simulink model "number"  (R2018a)
settings: Solver=VariableStepAuto  StartTime=0.0  StopTime=10.0  RelTol=1e-3
libraries: simulink_extras x32
settings Model: Creator=Edoardo Debenedetti  LastModifiedBy=Edoardo Debenedetti

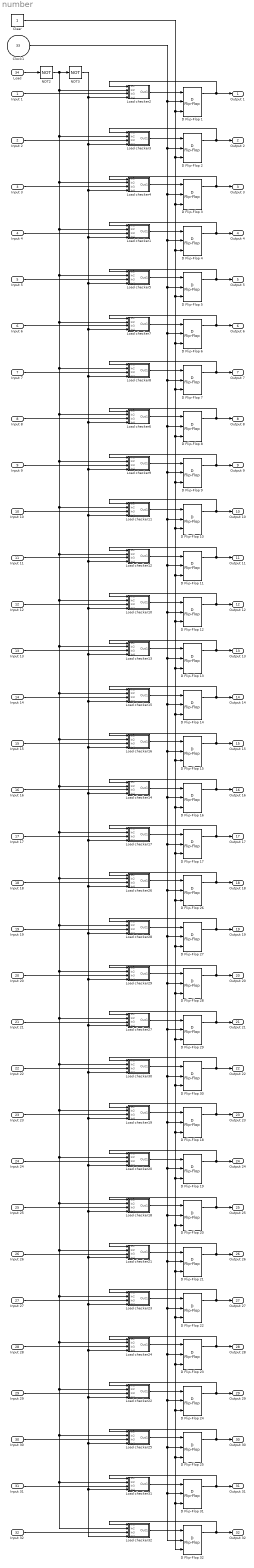
== system number ==
  Input 1 : Inport
  Input 2 : Inport  Port=2
  Input 3 : Inport  Port=3
  Input 4 : Inport  Port=4
  Input 5 : Inport  Port=5
  Input 6 : Inport  Port=6
  Input 7 : Inport  Port=7
  Input 8 : Inport  Port=8
  Input 9 : Inport  Port=9
  Input 10 : Inport  Port=10
  Input 11 : Inport  Port=11
  Input 12 : Inport  Port=12
  Input 13 : Inport  Port=13
  Input 14 : Inport  Port=14
  Input 15 : Inport  Port=15
  Input 16 : Inport  Port=16
  Input 17 : Inport  Port=17
  Input 18 : Inport  Port=18
  Input 19 : Inport  Port=19
  Input 20 : Inport  Port=20
  Input 21 : Inport  Port=21
  Input 22 : Inport  Port=22
  Input 23 : Inport  Port=23
  Input 24 : Inport  Port=24
  Input 25 : Inport  Port=25
  Input 26 : Inport  Port=26
  Input 27 : Inport  Port=27
  Input 28 : Inport  Port=28
  Input 29 : Inport  Port=29
  Input 30 : Inport  Port=30
  Input 31 : Inport  Port=31
  Input 32 : Inport  Port=32
  Clock1 : Inport  Port=33
  Load : Inport  Port=34
  Clear : Constant
  D Flip-Flop {1..32} (32 alike) : simulink_extras/Flip Flops/D Flip-Flop
      settings: SourceProductName=Simulink
  Load checker1 : Subsystem
  Load checker10 : Subsystem
  Load checker11 : Subsystem
  Load checker12 : Subsystem
  Load checker13 : Subsystem
  Load checker14 : Subsystem
  Load checker15 : Subsystem
  Load checker16 : Subsystem
  Load checker17 : Subsystem
  Load checker18 : Subsystem
  Load checker19 : Subsystem
  Load checker2 : Subsystem
  Load checker20 : Subsystem
  Load checker21 : Subsystem
  Load checker22 : Subsystem
  Load checker23 : Subsystem
  Load checker24 : Subsystem
  Load checker25 : Subsystem
  Load checker26 : Subsystem
  Load checker27 : Subsystem
  Load checker28 : Subsystem
  Load checker29 : Subsystem
  Load checker3 : Subsystem
  Load checker30 : Subsystem
  Load checker31 : Subsystem
  Load checker32 : Subsystem
  Load checker4 : Subsystem
  Load checker5 : Subsystem
  Load checker6 : Subsystem
  Load checker7 : Subsystem
  Load checker8 : Subsystem
  Load checker9 : Subsystem
  NOT2 : Logic  Operator=NOT  IconShape=distinctive  AllPortsSameDT=off  OutDataTypeStr=boolean
  NOT3 : Logic  Operator=NOT  IconShape=distinctive  AllPortsSameDT=off  OutDataTypeStr=boolean
  Output 1 : Outport
  Output 2 : Outport  Port=2
  Output 3 : Outport  Port=3
  Output 4 : Outport  Port=4
  Output 5 : Outport  Port=5
  Output 6 : Outport  Port=6
  Output 7 : Outport  Port=7
  Output 8 : Outport  Port=8
  Output 9 : Outport  Port=9
  Output 10 : Outport  Port=10
  Output 11 : Outport  Port=11
  Output 12 : Outport  Port=12
  Output 13 : Outport  Port=13
  Output 14 : Outport  Port=14
  Output 15 : Outport  Port=15
  Output 16 : Outport  Port=16
  Output 17 : Outport  Port=17
  Output 18 : Outport  Port=18
  Output 19 : Outport  Port=19
  Output 20 : Outport  Port=20
  Output 21 : Outport  Port=21
  Output 22 : Outport  Port=22
  Output 23 : Outport  Port=23
  Output 24 : Outport  Port=24
  Output 25 : Outport  Port=25
  Output 26 : Outport  Port=26
  Output 27 : Outport  Port=27
  Output 28 : Outport  Port=28
  Output 29 : Outport  Port=29
  Output 30 : Outport  Port=30
  Output 31 : Outport  Port=31
  Output 32 : Outport  Port=32
  wires:
  D Flip-Flop 1/1 -> Load checker2/1(In1), Output 1/1
  Load checker2/1(Out1) -> D Flip-Flop 1/1
  Input 1/1 -> Load checker2/3(In3)
  Load/1 -> NOT2/1
  Load checker3/1(Out1) -> D Flip-Flop 2/1
  D Flip-Flop 2/1 -> Load checker3/1(In1), Output 2/1
  Input 2/1 -> Load checker3/3(In3)
  Input 3/1 -> Load checker4/3(In3)
  D Flip-Flop 3/1 -> Output 3/1, Load checker4/1(In1)
  Load checker4/1(Out1) -> D Flip-Flop 3/1
  Load checker5/1(Out1) -> D Flip-Flop 5/1
  D Flip-Flop 5/1 -> Load checker5/1(In1), Output 5/1
  Input 5/1 -> Load checker5/3(In3)
  Input 4/1 -> Load checker1/3(In3)
  D Flip-Flop 4/1 -> Output 4/1, Load checker1/1(In1)
  Load checker1/1(Out1) -> D Flip-Flop 4/1
  Load checker6/1(Out1) -> D Flip-Flop 8/1
  D Flip-Flop 8/1 -> Load checker6/1(In1), Output 8/1
  Input 8/1 -> Load checker6/3(In3)
  Input 9/1 -> Load checker9/3(In3)
  D Flip-Flop 9/1 -> Output 9/1, Load checker9/1(In1)
  Load checker9/1(Out1) -> D Flip-Flop 9/1
  Load checker8/1(Out1) -> D Flip-Flop 7/1
  D Flip-Flop 7/1 -> Load checker8/1(In1), Output 7/1
  Input 7/1 -> Load checker8/3(In3)
  Input 6/1 -> Load checker7/3(In3)
  D Flip-Flop 6/1 -> Output 6/1, Load checker7/1(In1)
  Load checker7/1(Out1) -> D Flip-Flop 6/1
  Load checker15/1(Out1) -> D Flip-Flop 14/1
  D Flip-Flop 14/1 -> Load checker15/1(In1), Output 14/1
  Input 14/1 -> Load checker15/3(In3)
  Input 15/1 -> Load checker16/3(In3)
  D Flip-Flop 15/1 -> Output 15/1, Load checker16/1(In1)
  Load checker16/1(Out1) -> D Flip-Flop 15/1
  Load checker17/1(Out1) -> D Flip-Flop 17/1
  D Flip-Flop 17/1 -> Load checker17/1(In1), Output 17/1
  Input 17/1 -> Load checker17/3(In3)
  Input 16/1 -> Load checker14/3(In3)
  D Flip-Flop 16/1 -> Output 16/1, Load checker14/1(In1)
  Load checker14/1(Out1) -> D Flip-Flop 16/1
  Load checker10/1(Out1) -> D Flip-Flop 12/1
  D Flip-Flop 12/1 -> Load checker10/1(In1), Output 12/1
  Input 12/1 -> Load checker10/3(In3)
  Input 13/1 -> Load checker13/3(In3)
  D Flip-Flop 13/1 -> Output 13/1, Load checker13/1(In1)
  Load checker13/1(Out1) -> D Flip-Flop 13/1
  Load checker12/1(Out1) -> D Flip-Flop 11/1
  D Flip-Flop 11/1 -> Load checker12/1(In1), Output 11/1
  Input 11/1 -> Load checker12/3(In3)
  Input 10/1 -> Load checker11/3(In3)
  D Flip-Flop 10/1 -> Output 10/1, Load checker11/1(In1)
  Load checker11/1(Out1) -> D Flip-Flop 10/1
  Load checker19/1(Out1) -> D Flip-Flop 18/1
  D Flip-Flop 18/1 -> Load checker19/1(In1), Output 23/1
  Input 23/1 -> Load checker19/3(In3)
  Input 24/1 -> Load checker20/3(In3)
  D Flip-Flop 19/1 -> Output 24/1, Load checker20/1(In1)
  Load checker20/1(Out1) -> D Flip-Flop 19/1
  Load checker21/1(Out1) -> D Flip-Flop 21/1
  D Flip-Flop 21/1 -> Load checker21/1(In1), Output 26/1
  Input 26/1 -> Load checker21/3(In3)
  Input 25/1 -> Load checker18/3(In3)
  D Flip-Flop 20/1 -> Output 25/1, Load checker18/1(In1)
  Load checker18/1(Out1) -> D Flip-Flop 20/1
  Load checker22/1(Out1) -> D Flip-Flop 24/1
  D Flip-Flop 24/1 -> Load checker22/1(In1), Output 29/1
  Input 29/1 -> Load checker22/3(In3)
  Input 30/1 -> Load checker25/3(In3)
  D Flip-Flop 25/1 -> Output 30/1, Load checker25/1(In1)
  Load checker25/1(Out1) -> D Flip-Flop 25/1
  Load checker24/1(Out1) -> D Flip-Flop 23/1
  D Flip-Flop 23/1 -> Load checker24/1(In1), Output 28/1
  Input 28/1 -> Load checker24/3(In3)
  Input 27/1 -> Load checker23/3(In3)
  D Flip-Flop 22/1 -> Output 27/1, Load checker23/1(In1)
  Load checker23/1(Out1) -> D Flip-Flop 22/1
  Load checker28/1(Out1) -> D Flip-Flop 27/1
  D Flip-Flop 27/1 -> Load checker28/1(In1), Output 19/1
  Input 19/1 -> Load checker28/3(In3)
  Input 20/1 -> Load checker29/3(In3)
  D Flip-Flop 28/1 -> Output 20/1, Load checker29/1(In1)
  Load checker29/1(Out1) -> D Flip-Flop 28/1
  Load checker30/1(Out1) -> D Flip-Flop 30/1
  D Flip-Flop 30/1 -> Load checker30/1(In1), Output 22/1
  Input 22/1 -> Load checker30/3(In3)
  Input 21/1 -> Load checker27/3(In3)
  D Flip-Flop 29/1 -> Output 21/1, Load checker27/1(In1)
  Load checker27/1(Out1) -> D Flip-Flop 29/1
  Input 18/1 -> Load checker26/3(In3)
  D Flip-Flop 26/1 -> Output 18/1, Load checker26/1(In1)
  Load checker26/1(Out1) -> D Flip-Flop 26/1
  Clear/1 -> D Flip-Flop 10/3, D Flip-Flop 11/3, D Flip-Flop 12/3, D Flip-Flop 13/3, D Flip-Flop 14/3, D Flip-Flop 15/3, D Flip-Flop 16/3, D Flip-Flop 26/3, D Flip-Flop 27/3, D Flip-Flop 28/3, D Flip-Flop 29/3, D Flip-Flop 30/3, D Flip-Flop 31/3, D Flip-Flop 32/3, D Flip-Flop 25/3, D Flip-Flop 24/3, D Flip-Flop 23/3, D Flip-Flop 22/3, D Flip-Flop 21/3, D Flip-Flop 20/3, D Flip-Flop 19/3, D Flip-Flop 18/3, D Flip-Flop 17/3, D Flip-Flop 9/3, D Flip-Flop 8/3, D Flip-Flop 7/3, D Flip-Flop 6/3, D Flip-Flop 5/3, D Flip-Flop 4/3, D Flip-Flop 3/3, D Flip-Flop 2/3, D Flip-Flop 1/3
  Load checker32/1(Out1) -> D Flip-Flop 32/1
  D Flip-Flop 32/1 -> Load checker32/1(In1), Output 32/1
  NOT2/1 -> Load checker7/2(In2), Load checker8/2(In2), Load checker11/2(In2), Load checker12/2(In2), Load checker10/2(In2), Load checker13/2(In2), Load checker14/2(In2), Load checker26/2(In2), Load checker27/2(In2), Load checker30/2(In2), Load checker23/2(In2), Load checker24/2(In2), Load checker31/2(In2), Load checker32/2(In2), Load checker25/2(In2), Load checker22/2(In2), Load checker21/2(In2), Load checker18/2(In2), Load checker20/2(In2), Load checker19/2(In2), Load checker29/2(In2), Load checker28/2(In2), Load checker17/2(In2), Load checker16/2(In2), Load checker15/2(In2), Load checker9/2(In2), Load checker6/2(In2), Load checker5/2(In2), Load checker1/2(In2), Load checker4/2(In2), Load checker3/2(In2), Load checker2/2(In2), NOT3/1
  NOT3/1 -> Load checker1/4(In4), Load checker7/4(In4), Load checker8/4(In4), Load checker11/4(In4), Load checker12/4(In4), Load checker13/4(In4), Load checker14/4(In4), Load checker26/4(In4), Load checker27/4(In4), Load checker30/4(In4), Load checker18/4(In4), Load checker23/4(In4), Load checker24/4(In4), Load checker31/4(In4), Load checker32/4(In4), Load checker25/4(In4), Load checker22/4(In4), Load checker21/4(In4), Load checker20/4(In4), Load checker19/4(In4), Load checker29/4(In4), Load checker28/4(In4), Load checker17/4(In4), Load checker16/4(In4), Load checker15/4(In4), Load checker10/4(In4), Load checker9/4(In4), Load checker6/4(In4), Load checker5/4(In4), Load checker4/4(In4), Load checker3/4(In4), Load checker2/4(In4)
  Input 32/1 -> Load checker32/3(In3)
  Clock1/1 -> D Flip-Flop 4/2, D Flip-Flop 6/2, D Flip-Flop 7/2, D Flip-Flop 10/2, D Flip-Flop 11/2, D Flip-Flop 13/2, D Flip-Flop 16/2, D Flip-Flop 26/2, D Flip-Flop 29/2, D Flip-Flop 30/2, D Flip-Flop 20/2, D Flip-Flop 22/2, D Flip-Flop 23/2, D Flip-Flop 31/2, D Flip-Flop 32/2, D Flip-Flop 25/2, D Flip-Flop 24/2, D Flip-Flop 21/2, D Flip-Flop 19/2, D Flip-Flop 18/2, D Flip-Flop 28/2, D Flip-Flop 27/2, D Flip-Flop 17/2, D Flip-Flop 15/2, D Flip-Flop 14/2, D Flip-Flop 12/2, D Flip-Flop 9/2, D Flip-Flop 8/2, D Flip-Flop 5/2, D Flip-Flop 3/2, D Flip-Flop 2/2, D Flip-Flop 1/2
  Input 31/1 -> Load checker31/3(In3)
  D Flip-Flop 31/1 -> Output 31/1, Load checker31/1(In1)
  Load checker31/1(Out1) -> D Flip-Flop 31/1

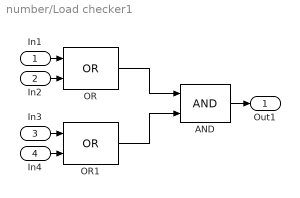
== system number/Load checker1 ==
  In1 : Inport
  In2 : Inport  Port=2
  In3 : Inport  Port=3
  In4 : Inport  Port=4
  AND : Logic  IconShape=distinctive  AllPortsSameDT=off  OutDataTypeStr=boolean
  OR : Logic  Operator=OR  IconShape=distinctive  AllPortsSameDT=off  OutDataTypeStr=boolean
  OR1 : Logic  Operator=OR  IconShape=distinctive  AllPortsSameDT=off  OutDataTypeStr=boolean
  Out1 : Outport
  wires:
  AND/1 -> Out1/1
  In2/1 -> OR/2
  In3/1 -> OR1/1
  In1/1 -> OR/1
  In4/1 -> OR1/2
  OR1/1 -> AND/2
  OR/1 -> AND/1

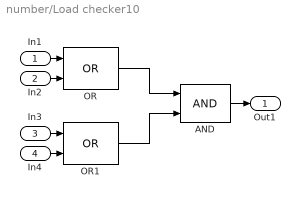
== system number/Load checker10 ==
  In1 : Inport
  In2 : Inport  Port=2
  In3 : Inport  Port=3
  In4 : Inport  Port=4
  AND : Logic  IconShape=distinctive  AllPortsSameDT=off  OutDataTypeStr=boolean
  OR : Logic  Operator=OR  IconShape=distinctive  AllPortsSameDT=off  OutDataTypeStr=boolean
  OR1 : Logic  Operator=OR  IconShape=distinctive  AllPortsSameDT=off  OutDataTypeStr=boolean
  Out1 : Outport
  wires:
  OR/1 -> AND/1
  OR1/1 -> AND/2
  In4/1 -> OR1/2
  In1/1 -> OR/1
  In3/1 -> OR1/1
  In2/1 -> OR/2
  AND/1 -> Out1/1

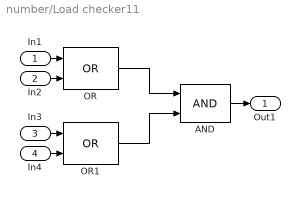
== system number/Load checker11 ==
  In1 : Inport
  In2 : Inport  Port=2
  In3 : Inport  Port=3
  In4 : Inport  Port=4
  AND : Logic  IconShape=distinctive  AllPortsSameDT=off  OutDataTypeStr=boolean
  OR : Logic  Operator=OR  IconShape=distinctive  AllPortsSameDT=off  OutDataTypeStr=boolean
  OR1 : Logic  Operator=OR  IconShape=distinctive  AllPortsSameDT=off  OutDataTypeStr=boolean
  Out1 : Outport
  wires:
  AND/1 -> Out1/1
  In2/1 -> OR/2
  In3/1 -> OR1/1
  In1/1 -> OR/1
  In4/1 -> OR1/2
  OR1/1 -> AND/2
  OR/1 -> AND/1

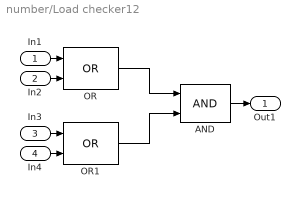
== system number/Load checker12 ==
  In1 : Inport
  In2 : Inport  Port=2
  In3 : Inport  Port=3
  In4 : Inport  Port=4
  AND : Logic  IconShape=distinctive  AllPortsSameDT=off  OutDataTypeStr=boolean
  OR : Logic  Operator=OR  IconShape=distinctive  AllPortsSameDT=off  OutDataTypeStr=boolean
  OR1 : Logic  Operator=OR  IconShape=distinctive  AllPortsSameDT=off  OutDataTypeStr=boolean
  Out1 : Outport
  wires:
  OR/1 -> AND/1
  OR1/1 -> AND/2
  In4/1 -> OR1/2
  In1/1 -> OR/1
  In3/1 -> OR1/1
  In2/1 -> OR/2
  AND/1 -> Out1/1

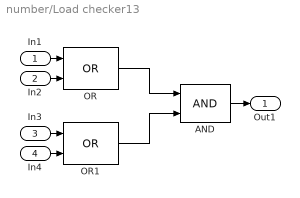
== system number/Load checker13 ==
  In1 : Inport
  In2 : Inport  Port=2
  In3 : Inport  Port=3
  In4 : Inport  Port=4
  AND : Logic  IconShape=distinctive  AllPortsSameDT=off  OutDataTypeStr=boolean
  OR : Logic  Operator=OR  IconShape=distinctive  AllPortsSameDT=off  OutDataTypeStr=boolean
  OR1 : Logic  Operator=OR  IconShape=distinctive  AllPortsSameDT=off  OutDataTypeStr=boolean
  Out1 : Outport
  wires:
  AND/1 -> Out1/1
  In2/1 -> OR/2
  In3/1 -> OR1/1
  In1/1 -> OR/1
  In4/1 -> OR1/2
  OR1/1 -> AND/2
  OR/1 -> AND/1

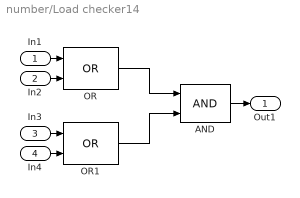
== system number/Load checker14 ==
  In1 : Inport
  In2 : Inport  Port=2
  In3 : Inport  Port=3
  In4 : Inport  Port=4
  AND : Logic  IconShape=distinctive  AllPortsSameDT=off  OutDataTypeStr=boolean
  OR : Logic  Operator=OR  IconShape=distinctive  AllPortsSameDT=off  OutDataTypeStr=boolean
  OR1 : Logic  Operator=OR  IconShape=distinctive  AllPortsSameDT=off  OutDataTypeStr=boolean
  Out1 : Outport
  wires:
  AND/1 -> Out1/1
  In2/1 -> OR/2
  In3/1 -> OR1/1
  In1/1 -> OR/1
  In4/1 -> OR1/2
  OR1/1 -> AND/2
  OR/1 -> AND/1

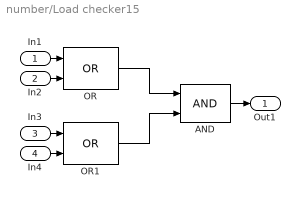
== system number/Load checker15 ==
  In1 : Inport
  In2 : Inport  Port=2
  In3 : Inport  Port=3
  In4 : Inport  Port=4
  AND : Logic  IconShape=distinctive  AllPortsSameDT=off  OutDataTypeStr=boolean
  OR : Logic  Operator=OR  IconShape=distinctive  AllPortsSameDT=off  OutDataTypeStr=boolean
  OR1 : Logic  Operator=OR  IconShape=distinctive  AllPortsSameDT=off  OutDataTypeStr=boolean
  Out1 : Outport
  wires:
  OR/1 -> AND/1
  OR1/1 -> AND/2
  In4/1 -> OR1/2
  In1/1 -> OR/1
  In3/1 -> OR1/1
  In2/1 -> OR/2
  AND/1 -> Out1/1

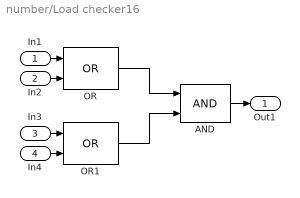
== system number/Load checker16 ==
  In1 : Inport
  In2 : Inport  Port=2
  In3 : Inport  Port=3
  In4 : Inport  Port=4
  AND : Logic  IconShape=distinctive  AllPortsSameDT=off  OutDataTypeStr=boolean
  OR : Logic  Operator=OR  IconShape=distinctive  AllPortsSameDT=off  OutDataTypeStr=boolean
  OR1 : Logic  Operator=OR  IconShape=distinctive  AllPortsSameDT=off  OutDataTypeStr=boolean
  Out1 : Outport
  wires:
  AND/1 -> Out1/1
  In2/1 -> OR/2
  In3/1 -> OR1/1
  In1/1 -> OR/1
  In4/1 -> OR1/2
  OR1/1 -> AND/2
  OR/1 -> AND/1

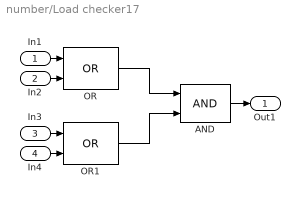
== system number/Load checker17 ==
  In1 : Inport
  In2 : Inport  Port=2
  In3 : Inport  Port=3
  In4 : Inport  Port=4
  AND : Logic  IconShape=distinctive  AllPortsSameDT=off  OutDataTypeStr=boolean
  OR : Logic  Operator=OR  IconShape=distinctive  AllPortsSameDT=off  OutDataTypeStr=boolean
  OR1 : Logic  Operator=OR  IconShape=distinctive  AllPortsSameDT=off  OutDataTypeStr=boolean
  Out1 : Outport
  wires:
  OR/1 -> AND/1
  OR1/1 -> AND/2
  In4/1 -> OR1/2
  In1/1 -> OR/1
  In3/1 -> OR1/1
  In2/1 -> OR/2
  AND/1 -> Out1/1

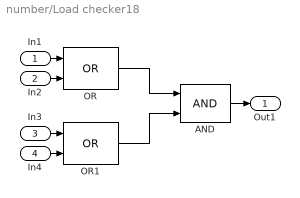
== system number/Load checker18 ==
  In1 : Inport
  In2 : Inport  Port=2
  In3 : Inport  Port=3
  In4 : Inport  Port=4
  AND : Logic  IconShape=distinctive  AllPortsSameDT=off  OutDataTypeStr=boolean
  OR : Logic  Operator=OR  IconShape=distinctive  AllPortsSameDT=off  OutDataTypeStr=boolean
  OR1 : Logic  Operator=OR  IconShape=distinctive  AllPortsSameDT=off  OutDataTypeStr=boolean
  Out1 : Outport
  wires:
  AND/1 -> Out1/1
  In2/1 -> OR/2
  In3/1 -> OR1/1
  In1/1 -> OR/1
  In4/1 -> OR1/2
  OR1/1 -> AND/2
  OR/1 -> AND/1

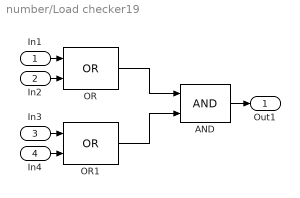
== system number/Load checker19 ==
  In1 : Inport
  In2 : Inport  Port=2
  In3 : Inport  Port=3
  In4 : Inport  Port=4
  AND : Logic  IconShape=distinctive  AllPortsSameDT=off  OutDataTypeStr=boolean
  OR : Logic  Operator=OR  IconShape=distinctive  AllPortsSameDT=off  OutDataTypeStr=boolean
  OR1 : Logic  Operator=OR  IconShape=distinctive  AllPortsSameDT=off  OutDataTypeStr=boolean
  Out1 : Outport
  wires:
  OR/1 -> AND/1
  OR1/1 -> AND/2
  In4/1 -> OR1/2
  In1/1 -> OR/1
  In3/1 -> OR1/1
  In2/1 -> OR/2
  AND/1 -> Out1/1

== system number/Load checker2 ==
  In1 : Inport
  In2 : Inport  Port=2
  In3 : Inport  Port=3
  In4 : Inport  Port=4
  AND : Logic  IconShape=distinctive  AllPortsSameDT=off  OutDataTypeStr=boolean
  OR : Logic  Operator=OR  IconShape=distinctive  AllPortsSameDT=off  OutDataTypeStr=boolean
  OR1 : Logic  Operator=OR  IconShape=distinctive  AllPortsSameDT=off  OutDataTypeStr=boolean
  Out1 : Outport
  wires:
  OR/1 -> AND/1
  OR1/1 -> AND/2
  In4/1 -> OR1/2
  In1/1 -> OR/1
  In3/1 -> OR1/1
  In2/1 -> OR/2
  AND/1 -> Out1/1

== system number/Load checker20 ==
  In1 : Inport
  In2 : Inport  Port=2
  In3 : Inport  Port=3
  In4 : Inport  Port=4
  AND : Logic  IconShape=distinctive  AllPortsSameDT=off  OutDataTypeStr=boolean
  OR : Logic  Operator=OR  IconShape=distinctive  AllPortsSameDT=off  OutDataTypeStr=boolean
  OR1 : Logic  Operator=OR  IconShape=distinctive  AllPortsSameDT=off  OutDataTypeStr=boolean
  Out1 : Outport
  wires:
  AND/1 -> Out1/1
  In2/1 -> OR/2
  In3/1 -> OR1/1
  In1/1 -> OR/1
  In4/1 -> OR1/2
  OR1/1 -> AND/2
  OR/1 -> AND/1

== system number/Load checker21 ==
  In1 : Inport
  In2 : Inport  Port=2
  In3 : Inport  Port=3
  In4 : Inport  Port=4
  AND : Logic  IconShape=distinctive  AllPortsSameDT=off  OutDataTypeStr=boolean
  OR : Logic  Operator=OR  IconShape=distinctive  AllPortsSameDT=off  OutDataTypeStr=boolean
  OR1 : Logic  Operator=OR  IconShape=distinctive  AllPortsSameDT=off  OutDataTypeStr=boolean
  Out1 : Outport
  wires:
  OR/1 -> AND/1
  OR1/1 -> AND/2
  In4/1 -> OR1/2
  In1/1 -> OR/1
  In3/1 -> OR1/1
  In2/1 -> OR/2
  AND/1 -> Out1/1

== system number/Load checker22 ==
  In1 : Inport
  In2 : Inport  Port=2
  In3 : Inport  Port=3
  In4 : Inport  Port=4
  AND : Logic  IconShape=distinctive  AllPortsSameDT=off  OutDataTypeStr=boolean
  OR : Logic  Operator=OR  IconShape=distinctive  AllPortsSameDT=off  OutDataTypeStr=boolean
  OR1 : Logic  Operator=OR  IconShape=distinctive  AllPortsSameDT=off  OutDataTypeStr=boolean
  Out1 : Outport
  wires:
  OR/1 -> AND/1
  OR1/1 -> AND/2
  In4/1 -> OR1/2
  In1/1 -> OR/1
  In3/1 -> OR1/1
  In2/1 -> OR/2
  AND/1 -> Out1/1

== system number/Load checker23 ==
  In1 : Inport
  In2 : Inport  Port=2
  In3 : Inport  Port=3
  In4 : Inport  Port=4
  AND : Logic  IconShape=distinctive  AllPortsSameDT=off  OutDataTypeStr=boolean
  OR : Logic  Operator=OR  IconShape=distinctive  AllPortsSameDT=off  OutDataTypeStr=boolean
  OR1 : Logic  Operator=OR  IconShape=distinctive  AllPortsSameDT=off  OutDataTypeStr=boolean
  Out1 : Outport
  wires:
  AND/1 -> Out1/1
  In2/1 -> OR/2
  In3/1 -> OR1/1
  In1/1 -> OR/1
  In4/1 -> OR1/2
  OR1/1 -> AND/2
  OR/1 -> AND/1

== system number/Load checker24 ==
  In1 : Inport
  In2 : Inport  Port=2
  In3 : Inport  Port=3
  In4 : Inport  Port=4
  AND : Logic  IconShape=distinctive  AllPortsSameDT=off  OutDataTypeStr=boolean
  OR : Logic  Operator=OR  IconShape=distinctive  AllPortsSameDT=off  OutDataTypeStr=boolean
  OR1 : Logic  Operator=OR  IconShape=distinctive  AllPortsSameDT=off  OutDataTypeStr=boolean
  Out1 : Outport
  wires:
  OR/1 -> AND/1
  OR1/1 -> AND/2
  In4/1 -> OR1/2
  In1/1 -> OR/1
  In3/1 -> OR1/1
  In2/1 -> OR/2
  AND/1 -> Out1/1

== system number/Load checker25 ==
  In1 : Inport
  In2 : Inport  Port=2
  In3 : Inport  Port=3
  In4 : Inport  Port=4
  AND : Logic  IconShape=distinctive  AllPortsSameDT=off  OutDataTypeStr=boolean
  OR : Logic  Operator=OR  IconShape=distinctive  AllPortsSameDT=off  OutDataTypeStr=boolean
  OR1 : Logic  Operator=OR  IconShape=distinctive  AllPortsSameDT=off  OutDataTypeStr=boolean
  Out1 : Outport
  wires:
  AND/1 -> Out1/1
  In2/1 -> OR/2
  In3/1 -> OR1/1
  In1/1 -> OR/1
  In4/1 -> OR1/2
  OR1/1 -> AND/2
  OR/1 -> AND/1

== system number/Load checker26 ==
  In1 : Inport
  In2 : Inport  Port=2
  In3 : Inport  Port=3
  In4 : Inport  Port=4
  AND : Logic  IconShape=distinctive  AllPortsSameDT=off  OutDataTypeStr=boolean
  OR : Logic  Operator=OR  IconShape=distinctive  AllPortsSameDT=off  OutDataTypeStr=boolean
  OR1 : Logic  Operator=OR  IconShape=distinctive  AllPortsSameDT=off  OutDataTypeStr=boolean
  Out1 : Outport
  wires:
  AND/1 -> Out1/1
  In2/1 -> OR/2
  In3/1 -> OR1/1
  In1/1 -> OR/1
  In4/1 -> OR1/2
  OR1/1 -> AND/2
  OR/1 -> AND/1

== system number/Load checker27 ==
  In1 : Inport
  In2 : Inport  Port=2
  In3 : Inport  Port=3
  In4 : Inport  Port=4
  AND : Logic  IconShape=distinctive  AllPortsSameDT=off  OutDataTypeStr=boolean
  OR : Logic  Operator=OR  IconShape=distinctive  AllPortsSameDT=off  OutDataTypeStr=boolean
  OR1 : Logic  Operator=OR  IconShape=distinctive  AllPortsSameDT=off  OutDataTypeStr=boolean
  Out1 : Outport
  wires:
  AND/1 -> Out1/1
  In2/1 -> OR/2
  In3/1 -> OR1/1
  In1/1 -> OR/1
  In4/1 -> OR1/2
  OR1/1 -> AND/2
  OR/1 -> AND/1

== system number/Load checker28 ==
  In1 : Inport
  In2 : Inport  Port=2
  In3 : Inport  Port=3
  In4 : Inport  Port=4
  AND : Logic  IconShape=distinctive  AllPortsSameDT=off  OutDataTypeStr=boolean
  OR : Logic  Operator=OR  IconShape=distinctive  AllPortsSameDT=off  OutDataTypeStr=boolean
  OR1 : Logic  Operator=OR  IconShape=distinctive  AllPortsSameDT=off  OutDataTypeStr=boolean
  Out1 : Outport
  wires:
  OR/1 -> AND/1
  OR1/1 -> AND/2
  In4/1 -> OR1/2
  In1/1 -> OR/1
  In3/1 -> OR1/1
  In2/1 -> OR/2
  AND/1 -> Out1/1

== system number/Load checker29 ==
  In1 : Inport
  In2 : Inport  Port=2
  In3 : Inport  Port=3
  In4 : Inport  Port=4
  AND : Logic  IconShape=distinctive  AllPortsSameDT=off  OutDataTypeStr=boolean
  OR : Logic  Operator=OR  IconShape=distinctive  AllPortsSameDT=off  OutDataTypeStr=boolean
  OR1 : Logic  Operator=OR  IconShape=distinctive  AllPortsSameDT=off  OutDataTypeStr=boolean
  Out1 : Outport
  wires:
  AND/1 -> Out1/1
  In2/1 -> OR/2
  In3/1 -> OR1/1
  In1/1 -> OR/1
  In4/1 -> OR1/2
  OR1/1 -> AND/2
  OR/1 -> AND/1

== system number/Load checker3 ==
  In1 : Inport
  In2 : Inport  Port=2
  In3 : Inport  Port=3
  In4 : Inport  Port=4
  AND : Logic  IconShape=distinctive  AllPortsSameDT=off  OutDataTypeStr=boolean
  OR : Logic  Operator=OR  IconShape=distinctive  AllPortsSameDT=off  OutDataTypeStr=boolean
  OR1 : Logic  Operator=OR  IconShape=distinctive  AllPortsSameDT=off  OutDataTypeStr=boolean
  Out1 : Outport
  wires:
  OR/1 -> AND/1
  OR1/1 -> AND/2
  In4/1 -> OR1/2
  In1/1 -> OR/1
  In3/1 -> OR1/1
  In2/1 -> OR/2
  AND/1 -> Out1/1

== system number/Load checker30 ==
  In1 : Inport
  In2 : Inport  Port=2
  In3 : Inport  Port=3
  In4 : Inport  Port=4
  AND : Logic  IconShape=distinctive  AllPortsSameDT=off  OutDataTypeStr=boolean
  OR : Logic  Operator=OR  IconShape=distinctive  AllPortsSameDT=off  OutDataTypeStr=boolean
  OR1 : Logic  Operator=OR  IconShape=distinctive  AllPortsSameDT=off  OutDataTypeStr=boolean
  Out1 : Outport
  wires:
  OR/1 -> AND/1
  OR1/1 -> AND/2
  In4/1 -> OR1/2
  In1/1 -> OR/1
  In3/1 -> OR1/1
  In2/1 -> OR/2
  AND/1 -> Out1/1

== system number/Load checker31 ==
  In1 : Inport
  In2 : Inport  Port=2
  In3 : Inport  Port=3
  In4 : Inport  Port=4
  AND : Logic  IconShape=distinctive  AllPortsSameDT=off  OutDataTypeStr=boolean
  OR : Logic  Operator=OR  IconShape=distinctive  AllPortsSameDT=off  OutDataTypeStr=boolean
  OR1 : Logic  Operator=OR  IconShape=distinctive  AllPortsSameDT=off  OutDataTypeStr=boolean
  Out1 : Outport
  wires:
  AND/1 -> Out1/1
  In2/1 -> OR/2
  In3/1 -> OR1/1
  In1/1 -> OR/1
  In4/1 -> OR1/2
  OR1/1 -> AND/2
  OR/1 -> AND/1

== system number/Load checker32 ==
  In1 : Inport
  In2 : Inport  Port=2
  In3 : Inport  Port=3
  In4 : Inport  Port=4
  AND : Logic  IconShape=distinctive  AllPortsSameDT=off  OutDataTypeStr=boolean
  OR : Logic  Operator=OR  IconShape=distinctive  AllPortsSameDT=off  OutDataTypeStr=boolean
  OR1 : Logic  Operator=OR  IconShape=distinctive  AllPortsSameDT=off  OutDataTypeStr=boolean
  Out1 : Outport
  wires:
  OR/1 -> AND/1
  OR1/1 -> AND/2
  In4/1 -> OR1/2
  In1/1 -> OR/1
  In3/1 -> OR1/1
  In2/1 -> OR/2
  AND/1 -> Out1/1

== system number/Load checker4 ==
  In1 : Inport
  In2 : Inport  Port=2
  In3 : Inport  Port=3
  In4 : Inport  Port=4
  AND : Logic  IconShape=distinctive  AllPortsSameDT=off  OutDataTypeStr=boolean
  OR : Logic  Operator=OR  IconShape=distinctive  AllPortsSameDT=off  OutDataTypeStr=boolean
  OR1 : Logic  Operator=OR  IconShape=distinctive  AllPortsSameDT=off  OutDataTypeStr=boolean
  Out1 : Outport
  wires:
  AND/1 -> Out1/1
  In2/1 -> OR/2
  In3/1 -> OR1/1
  In1/1 -> OR/1
  In4/1 -> OR1/2
  OR1/1 -> AND/2
  OR/1 -> AND/1

== system number/Load checker5 ==
  In1 : Inport
  In2 : Inport  Port=2
  In3 : Inport  Port=3
  In4 : Inport  Port=4
  AND : Logic  IconShape=distinctive  AllPortsSameDT=off  OutDataTypeStr=boolean
  OR : Logic  Operator=OR  IconShape=distinctive  AllPortsSameDT=off  OutDataTypeStr=boolean
  OR1 : Logic  Operator=OR  IconShape=distinctive  AllPortsSameDT=off  OutDataTypeStr=boolean
  Out1 : Outport
  wires:
  OR/1 -> AND/1
  OR1/1 -> AND/2
  In4/1 -> OR1/2
  In1/1 -> OR/1
  In3/1 -> OR1/1
  In2/1 -> OR/2
  AND/1 -> Out1/1

== system number/Load checker6 ==
  In1 : Inport
  In2 : Inport  Port=2
  In3 : Inport  Port=3
  In4 : Inport  Port=4
  AND : Logic  IconShape=distinctive  AllPortsSameDT=off  OutDataTypeStr=boolean
  OR : Logic  Operator=OR  IconShape=distinctive  AllPortsSameDT=off  OutDataTypeStr=boolean
  OR1 : Logic  Operator=OR  IconShape=distinctive  AllPortsSameDT=off  OutDataTypeStr=boolean
  Out1 : Outport
  wires:
  OR/1 -> AND/1
  OR1/1 -> AND/2
  In4/1 -> OR1/2
  In1/1 -> OR/1
  In3/1 -> OR1/1
  In2/1 -> OR/2
  AND/1 -> Out1/1

== system number/Load checker7 ==
  In1 : Inport
  In2 : Inport  Port=2
  In3 : Inport  Port=3
  In4 : Inport  Port=4
  AND : Logic  IconShape=distinctive  AllPortsSameDT=off  OutDataTypeStr=boolean
  OR : Logic  Operator=OR  IconShape=distinctive  AllPortsSameDT=off  OutDataTypeStr=boolean
  OR1 : Logic  Operator=OR  IconShape=distinctive  AllPortsSameDT=off  OutDataTypeStr=boolean
  Out1 : Outport
  wires:
  AND/1 -> Out1/1
  In2/1 -> OR/2
  In3/1 -> OR1/1
  In1/1 -> OR/1
  In4/1 -> OR1/2
  OR1/1 -> AND/2
  OR/1 -> AND/1

== system number/Load checker8 ==
  In1 : Inport
  In2 : Inport  Port=2
  In3 : Inport  Port=3
  In4 : Inport  Port=4
  AND : Logic  IconShape=distinctive  AllPortsSameDT=off  OutDataTypeStr=boolean
  OR : Logic  Operator=OR  IconShape=distinctive  AllPortsSameDT=off  OutDataTypeStr=boolean
  OR1 : Logic  Operator=OR  IconShape=distinctive  AllPortsSameDT=off  OutDataTypeStr=boolean
  Out1 : Outport
  wires:
  OR/1 -> AND/1
  OR1/1 -> AND/2
  In4/1 -> OR1/2
  In1/1 -> OR/1
  In3/1 -> OR1/1
  In2/1 -> OR/2
  AND/1 -> Out1/1

== system number/Load checker9 ==
  In1 : Inport
  In2 : Inport  Port=2
  In3 : Inport  Port=3
  In4 : Inport  Port=4
  AND : Logic  IconShape=distinctive  AllPortsSameDT=off  OutDataTypeStr=boolean
  OR : Logic  Operator=OR  IconShape=distinctive  AllPortsSameDT=off  OutDataTypeStr=boolean
  OR1 : Logic  Operator=OR  IconShape=distinctive  AllPortsSameDT=off  OutDataTypeStr=boolean
  Out1 : Outport
  wires:
  AND/1 -> Out1/1
  In2/1 -> OR/2
  In3/1 -> OR1/1
  In1/1 -> OR/1
  In4/1 -> OR1/2
  OR1/1 -> AND/2
  OR/1 -> AND/1
